simulink model "TestCVCalcBG"  (R2013a)
settings: Solver=ode45  StartTime=0.0  FixedStep=1e-4  RelTol=1e-3
values from neighbouring files (symbols this model uses):
  B = [B1;B2]    [GensetRespOptimiztion.m]    (also in GensetRespOptimiztionTorstein.m; Init8RTFLEX68D.m = 0.68; init_MVM.m = 0.127)
libraries: EngineSysteSubmodel x1
settings Model: Creator=yum  LastModifiedBy=yum
settings DataIOCC: ReturnWorkspaceOutputs=on

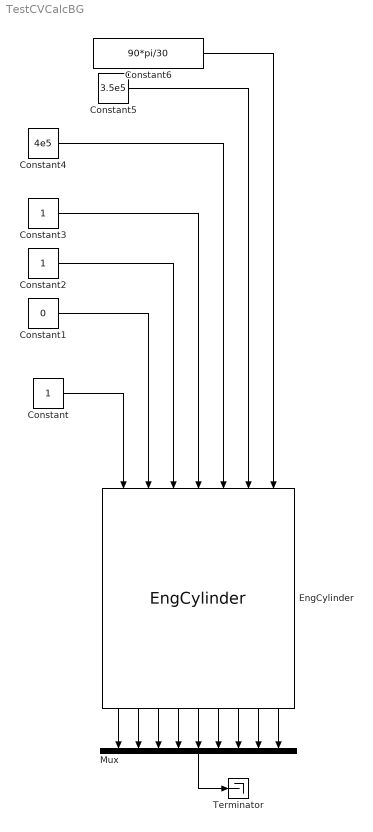
== system TestCVCalcBG ==
  Constant : Constant
  Constant1 : Constant  Value=0
  Constant2 : Constant
  Constant3 : Constant
  Constant4 : Constant  Value=4e5
  Constant5 : Constant  Value=3.5e5
  Constant6 : Constant  Value=90*pi/30
  EngCylinder : EngineSysteSubmodel/EngCylinder  fs=fs  nStroke=nStroke  hn=hn  nCyl=nCyl  iCyl=2  B=B  stroke=stroke  lambdaCrank=lambdaCrank  aCrank=aCrank  X=X  Y=Y  r=r  nPort=nPort  liftMax=liftMax  Dv=Dv  beta=beta  w=w  Dp=Dp  Ds=Ds  cAVVUpRef=cAVVUpRef  cAVVDownRef=cAVVDownRef  liftUpRef=liftUpRef  liftDownRef=liftDownRef  cAStartRef=cAStartRef  dCALiftUp=dCALiftUp  dCALiftDown=dCALiftDown  dCALiftTopRef=dCALiftTopRef  mCp=mCp  cCylHT=cCylHT  cAlpha=cAlpha  mqfCycMax=mqfCycMax  wiebePara=wiebePara  phi0=phi0  m0=mCyl0  E0=ECyl0  mb0=mbCyl0  V0=vCyl0  phi0A=phi0A  m0A=m0A  E0A=E0A  mb0A=mb0A  V0A=V0A
  Mux : Mux  Inputs=9
  Terminator : Terminator
  wires:
  Constant/1 -> EngCylinder/1
  Constant1/1 -> EngCylinder/2
  Constant2/1 -> EngCylinder/3
  Constant3/1 -> EngCylinder/4
  Constant4/1 -> EngCylinder/5
  Constant5/1 -> EngCylinder/6
  Constant6/1 -> EngCylinder/7
  EngCylinder/1 -> Mux/1
  EngCylinder/2 -> Mux/2
  EngCylinder/3 -> Mux/3
  EngCylinder/4 -> Mux/4
  EngCylinder/5 -> Mux/5
  EngCylinder/6 -> Mux/6
  EngCylinder/7 -> Mux/7
  EngCylinder/8 -> Mux/8
  EngCylinder/9 -> Mux/9
  Mux/1 -> Terminator/1
